simulink library "Time2Rotations"  (R2018b)
settings: Solver=VariableStepAuto  StartTime=0.0  StopTime=10.0  RelTol=1e-3
libraries: Rotations_Lib x1, Time x1
settings Model: Creator=IvanMachuca  LastModifiedBy=IvanMachuca

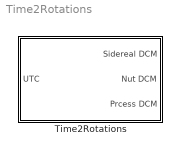
== system Time2Rotations ==
  "Time2Rotations " : Subsystem

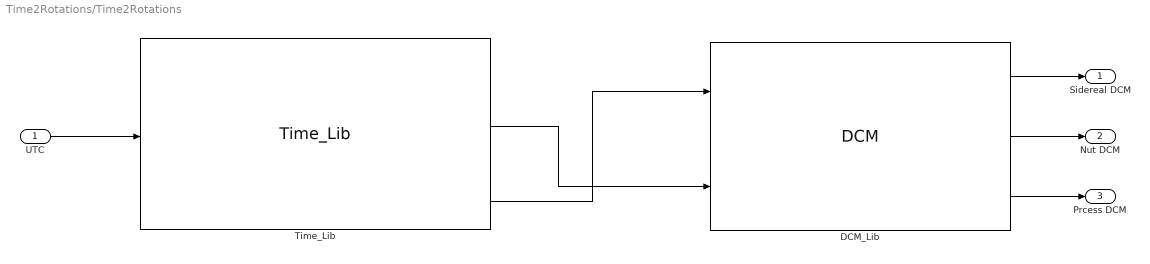
== system Time2Rotations/Time2Rotations  ==
  UTC : Inport
  "DCM_Lib " : Rotations_Lib/DCM   SystemSampleTime=-1
  "Time_Lib " : Time/Time_Lib    SystemSampleTime=-1
  Sidereal DCM : Outport
  "Nut DCM " : Outport  Port=2
  "Prcess DCM " : Outport  Port=3
  wires:
  "Time_Lib "/6 -> "DCM_Lib "/2
  "Time_Lib "/11 -> "DCM_Lib "/1
  UTC/1 -> "Time_Lib "/1
  "DCM_Lib "/1 -> Sidereal DCM/1
  "DCM_Lib "/2 -> "Nut DCM "/1
  "DCM_Lib "/3 -> "Prcess DCM "/1
